simulink model "final_simulation"  (R2023b)
settings: Solver=VariableStepAuto  StartTime=0.0  StopTime=300  RelTol=1e-3
values from neighbouring files (symbols this model uses):
  omega = v/R    [parameters.m]
  R = R1(3)    [parameters.m]
libraries: slpidlib x3
settings Model: Creator=swara  LastModifiedBy=muthu

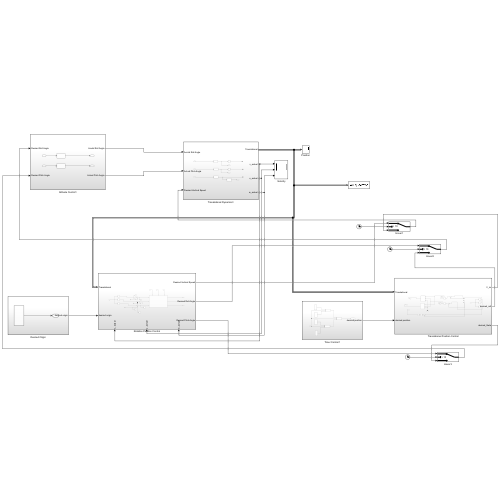
[thumbnail: Simulink's stored preview of the top-level diagram]
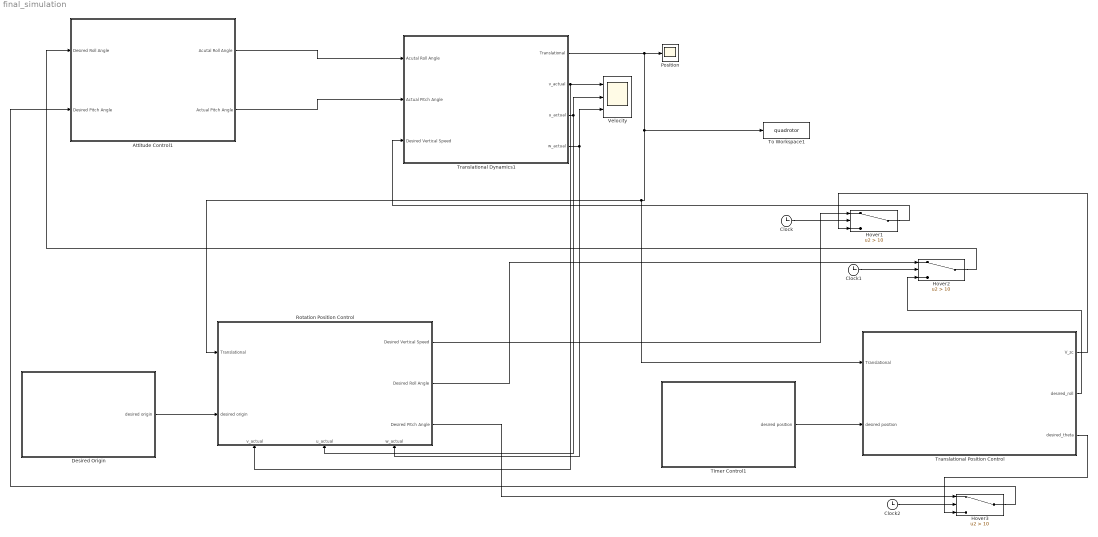
== system final_simulation ==
  Attitude Control1 : Subsystem
  Clock : Clock
  Clock1 : Clock
  Clock2 : Clock
  Desired Origin : Subsystem
  Hover1 : Switch  Criteria=u2 > Threshold  Threshold=10  SaturateOnIntegerOverflow=off  InputSameDT=off
  Hover2 : Switch  Criteria=u2 > Threshold  Threshold=10  SaturateOnIntegerOverflow=off  InputSameDT=off
  Hover3 : Switch  Criteria=u2 > Threshold  Threshold=10  SaturateOnIntegerOverflow=off  InputSameDT=off
  Position : Scope
  Rotation Position Control : Subsystem
      settings: PortSchema="{\"entries\":[{\"content\":{\"sides\":[{\"content\":{\"connectorIds\":[\"In1\",\"In2\"]},\"type\":\"ConnectorPlacement.EquallySpacedRectSide\",\"uuid\":\"b1b3e56e-3c02-4468-8ff7-9257e5b5e807\"},{\"content\":{\"connectorIds\":[\"Out1\",\"Out2\",\"Out3\"],\"side\":\"RIGHT\"},\"type\":\"ConnectorPlacement.EquallySpacedRectSide\",\"uuid\":\"224505eb-429b-4f4e-9eff-5e9145824b2b\"},{\"content\":{\"side\":\"TOP\"},\"type\":\"ConnectorPlacement.EquallySpacedRectSide\",\"uuid\":\"ae18805e-693a-4e7d-a4f9-b6e57170d54a\"},{\"content\":{\"connectorIds\":[\"In3\",\"In4\",\"In5\"],\"side\":\"BOTTOM\"},\"type\":\"ConnectorPlacement.EquallySpacedRectSide\",\"uuid\":\"834ddea8-6bbf-46e8-a21e-4332498dde7e\"}]},\"type\":\"ConnectorPlacement.EquallySpacedConnector\",\"uuid\":\"d1940db1-47fe-4a33-8f26-436ca695897e\"}],\"packageUris\":[\"http://schema.mathworks.com/mf0/Connector/R2020b\"],\"version\":\"1.0\"}"
  Timer Control1 : Subsystem
  To Workspace1 : ToWorkspace  VariableName=quadrotor  SampleTime=-1
  Translational Dynamics1 : Subsystem
  Translational Position Control : Subsystem
  Velocity : Scope  NumInputPorts=3
  wires:
  Attitude Control1/2(Actual Pitch Angle) -> Translational Dynamics1/2(Actual Pitch Angle)
  Translational Dynamics1/2(v_actual) -> Rotation Position Control/3(v_actual), Velocity/1
  Translational Dynamics1/3(u_actual) -> Rotation Position Control/4(u_actual), Velocity/2
  Translational Dynamics1/4(w_actual) -> Rotation Position Control/5(w_actual), Velocity/3
  Translational Dynamics1/1(Translational) -> Position/1, To Workspace1/1, Translational Position Control/1(Translational), Rotation Position Control/1(Translational)
  Attitude Control1/1(Acutal Roll Angle) -> Translational Dynamics1/1(Acutal Roll Angle)
  Desired Origin/1(desired origin) -> Rotation Position Control/2(desired origin)
  Translational Position Control/1(V_zc) -> Hover1/3
  Rotation Position Control/1(Desired Vertical Speed) -> Hover1/1
  Clock/1 -> Hover1/2
  Translational Position Control/2(desired_roll) -> Hover2/3
  Hover2/1 -> Attitude Control1/1(Desired Roll Angle)
  Rotation Position Control/2(Desired Roll Angle) -> Hover2/1
  Clock1/1 -> Hover2/2
  Translational Position Control/3(desired_theta) -> Hover3/3
  Rotation Position Control/3(Desired Pitch Angle) -> Hover3/1
  Clock2/1 -> Hover3/2
  Hover3/1 -> Attitude Control1/2(Desired Pitch Angle)
  Hover1/1 -> Translational Dynamics1/3(Desired Vertical Speed)
  Timer Control1/1(desired position) -> Translational Position Control/2(desired position)

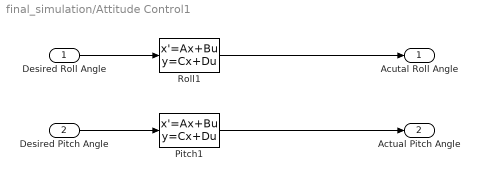
== system final_simulation/Attitude Control1 ==
  Desired Roll Angle : Inport
  Desired Pitch Angle : Inport  Port=2
  Pitch1 : StateSpace  A=[-3.9784 -2.9796; 4 0]  B=[2;0]  C=[1.2569 0.6083]  D=[0]  InitialCondition=0
  Roll1 : StateSpace  A=[-4.2683 -3.1716; 4 0]  B=[2;0]  C=[0.7417 0.4405]  D=[0]  InitialCondition=0
  Acutal Roll Angle : Outport
  Actual Pitch Angle : Outport  Port=2
  wires:
  Pitch1/1 -> Actual Pitch Angle/1
  Desired Pitch Angle/1 -> Pitch1/1
  Roll1/1 -> Acutal Roll Angle/1
  Desired Roll Angle/1 -> Roll1/1

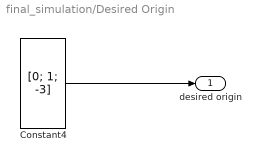
== system final_simulation/Desired Origin ==
  Constant4 : Constant  Value=[0; 1; -3]  VectorParams1D=off
  desired origin : Outport
  wires:
  Constant4/1 -> desired origin/1

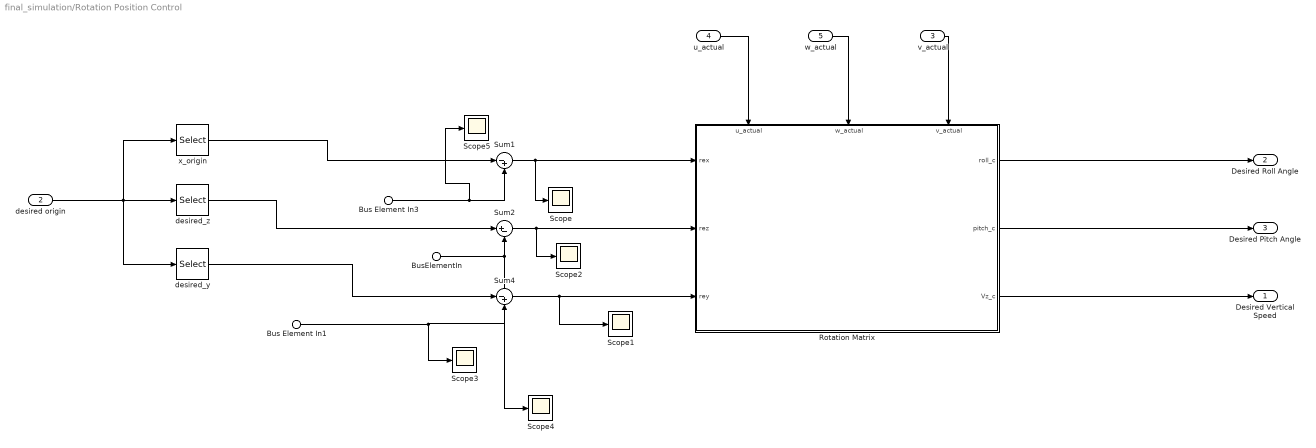
== system final_simulation/Rotation Position Control ==
  Bus Element In3 : Inport  PortName=Translational  Element=x_actual
  Bus Element In1 : Inport  PortName=Translational  Element=y_actual
  BusElementIn : Inport  PortName=Translational  Element=z_actual
  desired origin : Inport  Port=2
  v_actual : Inport  Port=3
  u_actual : Inport  Port=4
  w_actual : Inport  Port=5
  Rotation Matrix : Subsystem
      settings: PortSchema="{\"entries\":[{\"content\":{\"sides\":[{\"content\":{\"connectorIds\":[\"In1\",\"In2\",\"In3\"]},\"type\":\"ConnectorPlacement.EquallySpacedRectSide\",\"uuid\":\"851a648d-3d1b-4670-bb4b-4c1955b2d06c\"},{\"content\":{\"connectorIds\":[\"Out1\",\"Out2\",\"Out3\"],\"side\":\"RIGHT\"},\"type\":\"ConnectorPlacement.EquallySpacedRectSide\",\"uuid\":\"65ea146c-4b0b-429e-8e5f-57ab875054bb\"},{\"content\":{\"connectorIds\":[\"In4\",\"In5\",\"In6\"],\"side\":\"TOP\"},\"type\":\"ConnectorPlacement.EquallySpacedRectSide\",\"uuid\":\"0e78a648-e7f5-443e-b826-3dd94fb81bb4\"}]},\"type\":\"ConnectorPlacement.EquallySpacedConnector\",\"uuid\":\"33f91bbb-2c3f-4173-9364-ab3cef05faeb\"}],\"packageUris\":[\"http://schema.mathworks.com/mf0/Connector/R2020b\"],\"version\":\"1.0\"}"
  Scope{,1..5} (6 alike) : Scope
  Sum1 : Sum  Inputs=|-+
  Sum2 : Sum  Inputs=|+-
  Sum4 : Sum  Inputs=|-+
  desired_y : Selector  InputPortWidth=3  IndexOptions=Index vector (dialog)  Indices=[2]  OutputSizes=1
  desired_z : Selector  InputPortWidth=3  IndexOptions=Index vector (dialog)  Indices=[3]  OutputSizes=1
  x_origin : Selector  InputPortWidth=3  IndexOptions=Index vector (dialog)  Indices=[1]  OutputSizes=1
  Desired Vertical Speed : Outport
  Desired Roll Angle : Outport  Port=2
  Desired Pitch Angle : Outport  Port=3
  wires:
  Sum4/1 -> Scope1/1, Rotation Matrix/3(rey)
  x_origin/1 -> Sum1/1
  desired_y/1 -> Sum4/1
  desired_z/1 -> Sum2/1
  Sum2/1 -> Scope2/1, Rotation Matrix/2(rez)
  Rotation Matrix/1(roll_c) -> Desired Roll Angle/1
  Rotation Matrix/2(pitch_c) -> Desired Pitch Angle/1
  Rotation Matrix/3(Vz_c) -> Desired Vertical Speed/1
  BusElementIn/1 -> Scope4/1, Sum2/2
  v_actual/1 -> Rotation Matrix/6(v_actual)
  u_actual/1 -> Rotation Matrix/4(u_actual)
  w_actual/1 -> Rotation Matrix/5(w_actual)
  Sum1/1 -> Scope/1, Rotation Matrix/1(rex)
  Bus Element In3/1 -> Scope5/1, Sum1/2
  Bus Element In1/1 -> Scope3/1, Sum4/2
  desired origin/1 -> x_origin/1, desired_z/1, desired_y/1

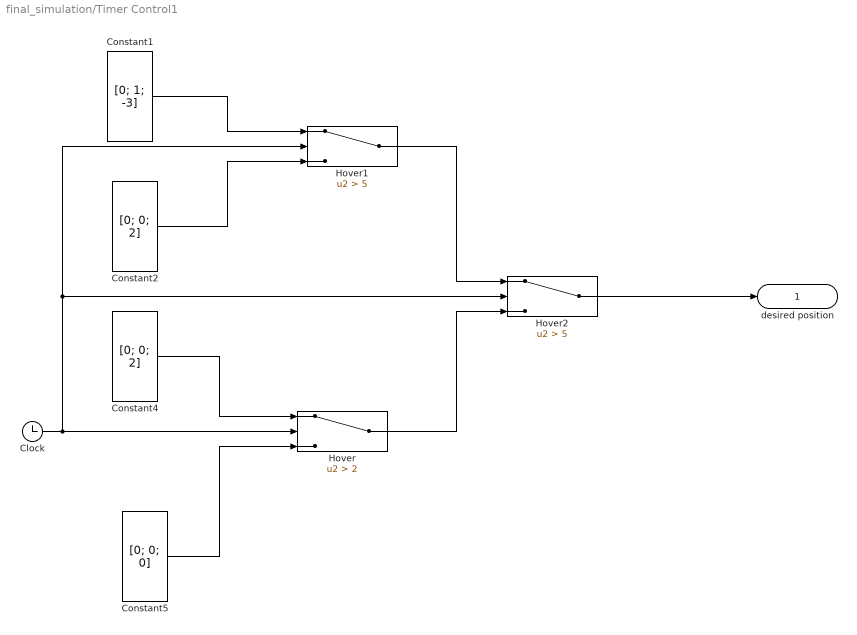
== system final_simulation/Timer Control1 ==
  Clock : Clock
  Constant1 : Constant  Value=[0; 1; -3]  VectorParams1D=off
  Constant2 : Constant  Value=[0; 0; 2]  VectorParams1D=off
  Constant4 : Constant  Value=[0; 0; 2]  VectorParams1D=off
  Constant5 : Constant  Value=[0; 0; 0]  VectorParams1D=off
  Hover : Switch  Criteria=u2 > Threshold  Threshold=2  SaturateOnIntegerOverflow=off  InputSameDT=off
  Hover1 : Switch  Criteria=u2 > Threshold  Threshold=5  SaturateOnIntegerOverflow=off  InputSameDT=off
  Hover2 : Switch  Criteria=u2 > Threshold  Threshold=5  SaturateOnIntegerOverflow=off  InputSameDT=off
  desired position : Outport
  wires:
  Hover1/1 -> Hover2/1
  Hover2/1 -> desired position/1
  Hover/1 -> Hover2/3
  Constant1/1 -> Hover1/1
  Constant2/1 -> Hover1/3
  Clock/1 -> Hover1/2, Hover2/2, Hover/2
  Constant5/1 -> Hover/3
  Constant4/1 -> Hover/1

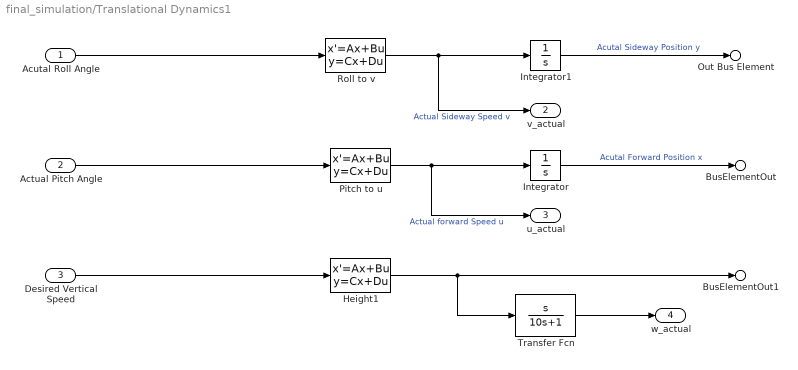
== system final_simulation/Translational Dynamics1 ==
  Acutal Roll Angle : Inport
  Actual Pitch Angle : Inport  Port=2
  Desired Vertical Speed : Inport  Port=3
  Height1 : StateSpace  A=[-5.82 -0.0000036046; 0.0000038147 0]  B=[1024;0]  C=[0.000014907 1319.1]  D=0  InitialCondition=0
  Integrator : Integrator
  Integrator1 : Integrator
  Pitch to u : StateSpace  A=[-0.665]  B=[2]  C=[-3.0772]  D=[0]  InitialCondition=0
  Roll to v : StateSpace  A=[-0.4596]  B=[2]  C=[2.3868]  D=[0]  InitialCondition=0
  Transfer Fcn : TransferFcn  Numerator=[1 0]  Denominator=[10 1]
  Out Bus Element : Outport  PortName=Translational  Element=y_actual
  BusElementOut : Outport  PortName=Translational  Element=x_actual
  BusElementOut1 : Outport  PortName=Translational  Element=z_actual
  v_actual : Outport  Port=2
  u_actual : Outport  Port=3
  w_actual : Outport  Port=4
  wires:
  Height1/1 -> Transfer Fcn/1, BusElementOut1/1
  Desired Vertical Speed/1 -> Height1/1
  Acutal Roll Angle/1 -> Roll to v/1
  Actual Pitch Angle/1 -> Pitch to u/1
  Integrator1/1 -> Out Bus Element/1  "Acutal Sideway Position y"
  Roll to v/1 -> v_actual/1, Integrator1/1  "Actual Sideway Speed v"
  Pitch to u/1 -> u_actual/1, Integrator/1  "Actual forward Speed u"
  Integrator/1 -> BusElementOut/1  "Acutal Forward Position x"
  Transfer Fcn/1 -> w_actual/1

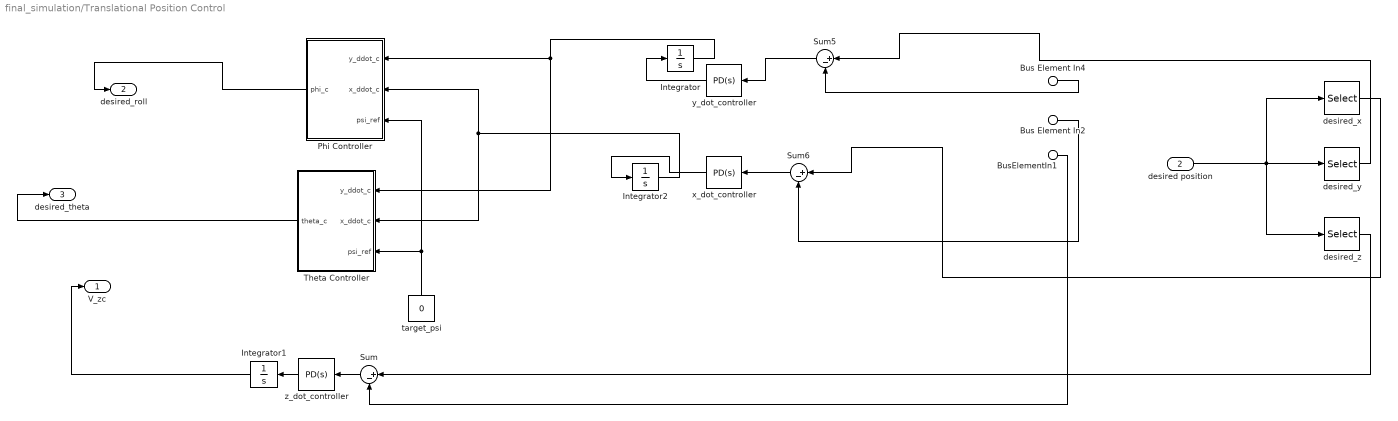
== system final_simulation/Translational Position Control ==
  Bus Element In2 : Inport  PortName=Translational  Element=x_actual
  Bus Element In4 : Inport  PortName=Translational  Element=y_actual
  BusElementIn1 : Inport  PortName=Translational  Element=z_actual
  desired position : Inport  Port=2
  Integrator : Integrator
  Integrator1 : Integrator
  Integrator2 : Integrator
  Phi Controller : Subsystem
  Sum : Sum  Inputs=|+-
  Sum5 : Sum  Inputs=|+-
  Sum6 : Sum  Inputs=|+-
  Theta Controller : Subsystem
  desired_x : Selector  InputPortWidth=3  IndexOptions=Index vector (dialog)  Indices=[1]  OutputSizes=1
  desired_y : Selector  InputPortWidth=3  IndexOptions=Index vector (dialog)  Indices=[2]  OutputSizes=1
  desired_z : Selector  InputPortWidth=3  IndexOptions=Index vector (dialog)  Indices=[3]  OutputSizes=1
  target_psi : Constant  Value=0
  x_dot_controller : slpidlib/PID Controller  Controller=PD  Form=Parallel  TimeDomain=Continuous-time  UseExternalTs=off  SampleTime=-1  IntegratorMethod=Forward Euler  FilterMethod=Forward Euler  ControllerParametersSource=internal  P=0.000973164818719708  I=10  UseKiTs=off  D=0.547582496129018  N=23.2094749491002  UseFilter=on  TunerSelectOption=Transfer Function Based (PID Tuner App)  InitialConditionSource=internal  InitialConditionForIntegrator=0  InitialConditionForFilter=0  DifferentiatorICPrevScaledInput=0  ExternalReset=none  TrackingMode=off  Kt=1  LimitOutput=off  SatLimitsSource=internal  UpperSaturationLimit=inf  LowerSaturationLimit=-inf  LinearizeAsGain=on  AntiWindupMode=none  Kb=1  LimitIntegrator=off  UpperIntegratorSaturationLimit=inf  LowerIntegratorSaturationLimit=-inf  POutMin=[]  POutMax=[]  IOutMin=[]  IOutMax=[]  DOutMin=[]  DOutMax=[]  NOutMin=[]  NOutMax=[]  SumOutMin=[]  SumOutMax=[]  SaturationOutMin=[]  SaturationOutMax=[]  PParamMin=[]  PParamMax=[]  IParamMin=[]  IParamMax=[]  DParamMin=[]  DParamMax=[]  NParamMin=[]  NParamMax=[]  KbParamMin=[]  KbParamMax=[]  KtParamMin=[]  KtParamMax=[]  KbOutMin=[]  KbOutMax=[]  KtOutMin=[]  KtOutMax=[]  IntegratorOutMin=[]  IntegratorOutMax=[]  FilterOutMin=[]  FilterOutMax=[]  SumI1OutMin=[]  SumI1OutMax=[]  SumI2OutMin=[]  SumI2OutMax=[]  SumI3OutMin=[]  SumI3OutMax=[]  SumI4OutMin=[]  SumI4OutMax=[]  SumDOutMin=[]  SumDOutMax=[]  DifferentiatorOutMin=[]  DifferentiatorOutMax=[]  FilterDiffOutCoefMin=[]  FilterDiffOutCoefMax=[]  ReciprocalOutMin=[]  ReciprocalOutMax=[]  SumDenOutMin=[]  SumDenOutMax=[]  SumNumOutMin=[]  SumNumOutMax=[]  DivideOutMin=[]  DivideOutMax=[]  UdiffTsProdOutMin=[]  UdiffTsProdOutMax=[]  NTsProdOutMin=[]  NTsProdOutMax=[]  UintegralTsProdOutMin=[]  UintegralTsProdOutMax=[]  UngainTsProdOutMin=[]  UngainTsProdOutMax=[]  ClampingZeroOutDataTypeStr=Inherit: Inherit via back propagation  ClampingZeroOutMin=[]  ClampingZeroOutMax=[]  FilterDenConstantOutDataTypeStr=Inherit: Inherit via back propagation  FilterDenConstantOutMin=[]  FilterDenConstantOutMax=[]  PCopyOutDataTypeStr=Inherit: Inherit via back propagation  PCopyOutMin=[]  PCopyOutMax=[]  NCopyOutDataTypeStr=Inherit: Inherit via back propagation  NCopyOutMin=[]  NCopyOutMax=[]  IntegratorContinuousStateAttributes=''  IntegratorStateMustResolveToSignalObject=off  IntegratorRTWStateStorageClass=Auto  FilterContinuousStateAttributes=''  FilterStateMustResolveToSignalObject=off  FilterRTWStateStorageClass=Auto  ParallelPVariant=InternalParameters  IdealPVariant=Disabled  IVariant=Disabled  DVariant=InternalParameters  IntegratorVariant=Disabled  SatVariant=Disabled  AWVariant=Disabled  PCopyVariant=Disabled  TRVariant=Disabled  FdbkBlocksVariant=Forward  IdealPFdbkVariant=Disabled  SatFdbkVariant=Disabled  DerivativeFilterVariant=ContFilter  NVariant=InternalParameters  NCopyVariant=Disabled  FilterICVariant=InternalICsFilter  IntegratorICVariant=Disabled  ExternalResetVariant=Disabled  TRSumVariant=Passthrough  SumFdbkVariant=Disabled  SumVariant=Sum_PD  TsampFilterVariant=InternalTs  TsampNgainVariant=Passthrough  TsampIntegralVariant=Disabled_SignalSpec  ExternalSaturationOutDataTypeStr=Inherit: Same as second input
  y_dot_controller : slpidlib/PID Controller  Controller=PD  Form=Parallel  TimeDomain=Continuous-time  UseExternalTs=off  SampleTime=-1  IntegratorMethod=Forward Euler  FilterMethod=Forward Euler  ControllerParametersSource=internal  P=0.390400736412338878  I=10  UseKiTs=off  D=0.400269327887123  N=13.0747973581782  UseFilter=on  TunerSelectOption=Transfer Function Based (PID Tuner App)  InitialConditionSource=internal  InitialConditionForIntegrator=0  InitialConditionForFilter=0  DifferentiatorICPrevScaledInput=0  ExternalReset=none  TrackingMode=off  Kt=1  LimitOutput=off  SatLimitsSource=internal  UpperSaturationLimit=inf  LowerSaturationLimit=-inf  LinearizeAsGain=on  AntiWindupMode=none  Kb=1  LimitIntegrator=off  UpperIntegratorSaturationLimit=inf  LowerIntegratorSaturationLimit=-inf  POutMin=[]  POutMax=[]  IOutMin=[]  IOutMax=[]  DOutMin=[]  DOutMax=[]  NOutMin=[]  NOutMax=[]  SumOutMin=[]  SumOutMax=[]  SaturationOutMin=[]  SaturationOutMax=[]  PParamMin=[]  PParamMax=[]  IParamMin=[]  IParamMax=[]  DParamMin=[]  DParamMax=[]  NParamMin=[]  NParamMax=[]  KbParamMin=[]  KbParamMax=[]  KtParamMin=[]  KtParamMax=[]  KbOutMin=[]  KbOutMax=[]  KtOutMin=[]  KtOutMax=[]  IntegratorOutMin=[]  IntegratorOutMax=[]  FilterOutMin=[]  FilterOutMax=[]  SumI1OutMin=[]  SumI1OutMax=[]  SumI2OutMin=[]  SumI2OutMax=[]  SumI3OutMin=[]  SumI3OutMax=[]  SumI4OutMin=[]  SumI4OutMax=[]  SumDOutMin=[]  SumDOutMax=[]  DifferentiatorOutMin=[]  DifferentiatorOutMax=[]  FilterDiffOutCoefMin=[]  FilterDiffOutCoefMax=[]  ReciprocalOutMin=[]  ReciprocalOutMax=[]  SumDenOutMin=[]  SumDenOutMax=[]  SumNumOutMin=[]  SumNumOutMax=[]  DivideOutMin=[]  DivideOutMax=[]  UdiffTsProdOutMin=[]  UdiffTsProdOutMax=[]  NTsProdOutMin=[]  NTsProdOutMax=[]  UintegralTsProdOutMin=[]  UintegralTsProdOutMax=[]  UngainTsProdOutMin=[]  UngainTsProdOutMax=[]  ClampingZeroOutDataTypeStr=Inherit: Inherit via back propagation  ClampingZeroOutMin=[]  ClampingZeroOutMax=[]  FilterDenConstantOutDataTypeStr=Inherit: Inherit via back propagation  FilterDenConstantOutMin=[]  FilterDenConstantOutMax=[]  PCopyOutDataTypeStr=Inherit: Inherit via back propagation  PCopyOutMin=[]  PCopyOutMax=[]  NCopyOutDataTypeStr=Inherit: Inherit via back propagation  NCopyOutMin=[]  NCopyOutMax=[]  IntegratorContinuousStateAttributes=''  IntegratorStateMustResolveToSignalObject=off  IntegratorRTWStateStorageClass=Auto  FilterContinuousStateAttributes=''  FilterStateMustResolveToSignalObject=off  FilterRTWStateStorageClass=Auto  ParallelPVariant=InternalParameters  IdealPVariant=Disabled  IVariant=Disabled  DVariant=InternalParameters  IntegratorVariant=Disabled  SatVariant=Disabled  AWVariant=Disabled  PCopyVariant=Disabled  TRVariant=Disabled  FdbkBlocksVariant=Forward  IdealPFdbkVariant=Disabled  SatFdbkVariant=Disabled  DerivativeFilterVariant=ContFilter  NVariant=InternalParameters  NCopyVariant=Disabled  FilterICVariant=InternalICsFilter  IntegratorICVariant=Disabled  ExternalResetVariant=Disabled  TRSumVariant=Passthrough  SumFdbkVariant=Disabled  SumVariant=Sum_PD  TsampFilterVariant=InternalTs  TsampNgainVariant=Passthrough  TsampIntegralVariant=Disabled_SignalSpec  ExternalSaturationOutDataTypeStr=Inherit: Same as second input
  z_dot_controller : slpidlib/PID Controller  Controller=PD  Form=Parallel  TimeDomain=Continuous-time  UseExternalTs=off  SampleTime=-1  IntegratorMethod=Forward Euler  FilterMethod=Forward Euler  ControllerParametersSource=internal  P=0.3  I=1  UseKiTs=off  D=3  N=100  UseFilter=on  TunerSelectOption=Transfer Function Based (PID Tuner App)  InitialConditionSource=internal  InitialConditionForIntegrator=0  InitialConditionForFilter=0  DifferentiatorICPrevScaledInput=0  ExternalReset=none  TrackingMode=off  Kt=1  LimitOutput=off  SatLimitsSource=internal  UpperSaturationLimit=inf  LowerSaturationLimit=-inf  LinearizeAsGain=on  AntiWindupMode=none  Kb=1  LimitIntegrator=off  UpperIntegratorSaturationLimit=inf  LowerIntegratorSaturationLimit=-inf  POutMin=[]  POutMax=[]  IOutMin=[]  IOutMax=[]  DOutMin=[]  DOutMax=[]  NOutMin=[]  NOutMax=[]  SumOutMin=[]  SumOutMax=[]  SaturationOutMin=[]  SaturationOutMax=[]  PParamMin=[]  PParamMax=[]  IParamMin=[]  IParamMax=[]  DParamMin=[]  DParamMax=[]  NParamMin=[]  NParamMax=[]  KbParamMin=[]  KbParamMax=[]  KtParamMin=[]  KtParamMax=[]  KbOutMin=[]  KbOutMax=[]  KtOutMin=[]  KtOutMax=[]  IntegratorOutMin=[]  IntegratorOutMax=[]  FilterOutMin=[]  FilterOutMax=[]  SumI1OutMin=[]  SumI1OutMax=[]  SumI2OutMin=[]  SumI2OutMax=[]  SumI3OutMin=[]  SumI3OutMax=[]  SumI4OutMin=[]  SumI4OutMax=[]  SumDOutMin=[]  SumDOutMax=[]  DifferentiatorOutMin=[]  DifferentiatorOutMax=[]  FilterDiffOutCoefMin=[]  FilterDiffOutCoefMax=[]  ReciprocalOutMin=[]  ReciprocalOutMax=[]  SumDenOutMin=[]  SumDenOutMax=[]  SumNumOutMin=[]  SumNumOutMax=[]  DivideOutMin=[]  DivideOutMax=[]  UdiffTsProdOutMin=[]  UdiffTsProdOutMax=[]  NTsProdOutMin=[]  NTsProdOutMax=[]  UintegralTsProdOutMin=[]  UintegralTsProdOutMax=[]  UngainTsProdOutMin=[]  UngainTsProdOutMax=[]  ClampingZeroOutDataTypeStr=Inherit: Inherit via back propagation  ClampingZeroOutMin=[]  ClampingZeroOutMax=[]  FilterDenConstantOutDataTypeStr=Inherit: Inherit via back propagation  FilterDenConstantOutMin=[]  FilterDenConstantOutMax=[]  PCopyOutDataTypeStr=Inherit: Inherit via back propagation  PCopyOutMin=[]  PCopyOutMax=[]  NCopyOutDataTypeStr=Inherit: Inherit via back propagation  NCopyOutMin=[]  NCopyOutMax=[]  IntegratorContinuousStateAttributes=''  IntegratorStateMustResolveToSignalObject=off  IntegratorRTWStateStorageClass=Auto  FilterContinuousStateAttributes=''  FilterStateMustResolveToSignalObject=off  FilterRTWStateStorageClass=Auto  ParallelPVariant=InternalParameters  IdealPVariant=Disabled  IVariant=Disabled  DVariant=InternalParameters  IntegratorVariant=Disabled  SatVariant=Disabled  AWVariant=Disabled  PCopyVariant=Disabled  TRVariant=Disabled  FdbkBlocksVariant=Forward  IdealPFdbkVariant=Disabled  SatFdbkVariant=Disabled  DerivativeFilterVariant=ContFilter  NVariant=InternalParameters  NCopyVariant=Disabled  FilterICVariant=InternalICsFilter  IntegratorICVariant=Disabled  ExternalResetVariant=Disabled  TRSumVariant=Passthrough  SumFdbkVariant=Disabled  SumVariant=Sum_PD  TsampFilterVariant=InternalTs  TsampNgainVariant=Passthrough  TsampIntegralVariant=Disabled_SignalSpec  ExternalSaturationOutDataTypeStr=Inherit: Same as second input
  V_zc : Outport
  desired_roll : Outport  Port=2
  desired_theta : Outport  Port=3
  wires:
  y_dot_controller/1 -> Integrator/1
  desired position/1 -> desired_z/1, desired_x/1, desired_y/1
  target_psi/1 -> Phi Controller/3(psi_ref), Theta Controller/3(psi_ref)
  z_dot_controller/1 -> Integrator1/1
  Sum5/1 -> y_dot_controller/1
  x_dot_controller/1 -> Integrator2/1
  Sum6/1 -> x_dot_controller/1
  Sum/1 -> z_dot_controller/1
  Bus Element In2/1 -> Sum6/2
  Integrator2/1 -> Theta Controller/2(x_ddot_c), Phi Controller/2(x_ddot_c)
  desired_y/1 -> Sum5/1
  Integrator/1 -> Theta Controller/1(y_ddot_c), Phi Controller/1(y_ddot_c)
  Bus Element In4/1 -> Sum5/2
  desired_x/1 -> Sum6/1
  desired_z/1 -> Sum/1
  BusElementIn1/1 -> Sum/2
  Phi Controller/1(phi_c) -> desired_roll/1
  Theta Controller/1(theta_c) -> desired_theta/1
  Integrator1/1 -> V_zc/1

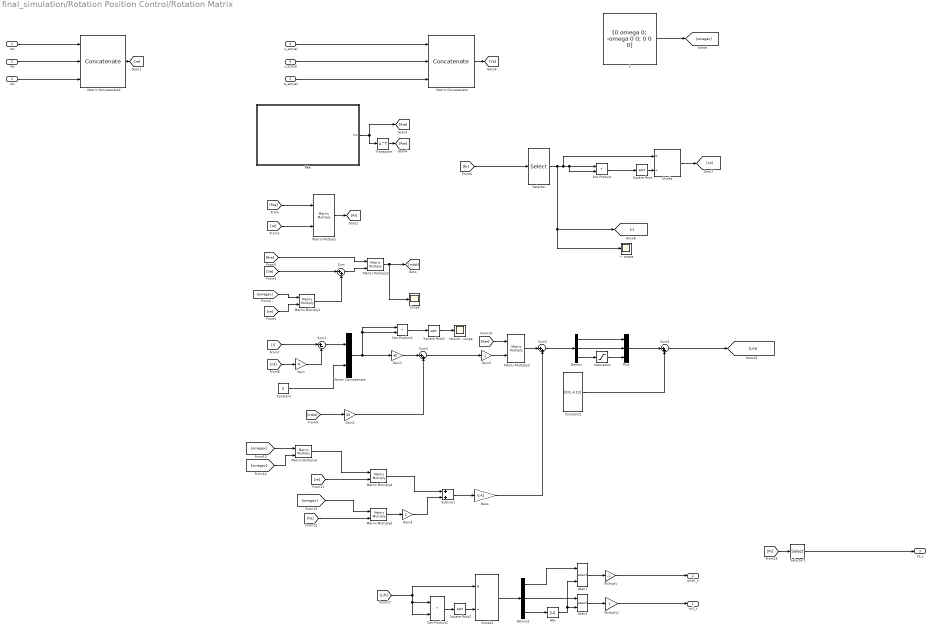
== system final_simulation/Rotation Position Control/Rotation Matrix ==
  rex : Inport
  rez : Inport  Port=2
  rey : Inport  Port=3
  u_actual : Inport  Port=4
  w_actual : Inport  Port=5
  v_actual : Inport  Port=6
  1 : Constant  Value=[0 omega 0; -omega 0 0; 0 0 0]  VectorParams1D=off
  Abs : Abs  SaturateOnIntegerOverflow=off
  Atan1 : Trigonometry  Operator=atan2
  Atan2 : Trigonometry  Operator=atan2
  Constant : Constant  Value=0
  Constant2 : Constant  Value=[0;0;-4.12]  VectorParams1D=off
  Demux : Demux  Outputs=3
  Demux1 : Demux  Outputs=3
  Divide : Product  Inputs=*/
  Divide1 : Product  Inputs=*/
  Dot Product : DotProduct  OutDataTypeStr=Inherit: Inherit via internal rule
  Dot Product1 : DotProduct  OutDataTypeStr=Inherit: Inherit via internal rule
  Dot Product2 : DotProduct  OutDataTypeStr=Inherit: Inherit via internal rule
  Gain : Gain  Gain=R
  Gain1 : Gain  Gain=40
  Gain2 : Gain  Gain=30
  Gain3 : Gain  Gain=-1
  Gain4 : Gain  Gain=2
  Mass : Gain  Gain=0.42
  Matrix Concatenate : Concatenate  NumInputs=3  Mode=Multidimensional array
  Matrix Concatenate2 : Concatenate  NumInputs=3  Mode=Multidimensional array
  Matrix Multiply{,1..6} (7 alike) : Product  Multiplication=Matrix(*)
  Multiply : Gain  Gain=-1
  Multiply1 : Gain
  Mux : Mux  Inputs=3
  RRe : Subsystem
  Saturation : Saturate
  Scope : Scope
  Selector : Selector  InputPortWidth=3  IndexOptions=Index vector (dialog)  Indices=[1 2]  OutputSizes=1
  Selector1 : Selector  InputPortWidth=3  IndexOptions=Index vector (dialog)  Indices=[3]  OutputSizes=1
  Square Root : Sqrt
  Square Root1 : Sqrt
  Square Root2 : Sqrt
  Subtract : Sum
  Sum{,2..4} (4 alike) : Sum  Inputs=|++
  Sum1 : Sum  Inputs=|+-
  Transpose : Math  Operator=transpose  SignedPower=on
  Vector Concatenate : Concatenate
  r - scope : Scope
  rdnorm - scope : Scope
  roll_c : Outport
  pitch_c : Outport  Port=2
  Vz_c : Outport  Port=3
  wires:
  rex/1 -> Matrix Concatenate2/1
  RRe/1(RdI) -> Transpose/1, [Rre]
  Transpose/1 -> [Rer]
  [Rre] -> Matrix Multiply/1
  [re] -> Matrix Multiply/2
  Matrix Multiply/1 -> [Rr]
  u_actual/1 -> Matrix Concatenate/1
  v_actual/1 -> Matrix Concatenate/2
  rey/1 -> Matrix Concatenate2/2
  Matrix Concatenate/1 -> [Ve]
  [omegax] -> Matrix Multiply1/1
  [re] -> Matrix Multiply1/2
  Matrix Multiply1/1 -> Sum/2
  [Ve] -> Sum/1
  Sum/1 -> Matrix Multiply2/2
  [Rre] -> Matrix Multiply2/1
  Matrix Multiply2/1 -> Scope/1, [rrdot]
  1/1 -> [omegax]
  Square Root/1 -> Divide/2
  Divide/1 -> [n2]
  [n2] -> Gain/1
  [r] -> Sum1/1
  Gain/1 -> Sum1/2
  Sum1/1 -> Vector Concatenate/1
  Constant/1 -> Vector Concatenate/2
  Vector Concatenate/1 -> Dot Product1/1, Dot Product1/2, Gain1/1
  Dot Product1/1 -> Square Root1/1
  [rrdot] -> Gain2/1
  Gain1/1 -> Sum2/1
  Gain2/1 -> Sum2/2
  Sum2/1 -> Gain3/1
  Gain3/1 -> Matrix Multiply3/2
  [Rer] -> Matrix Multiply3/1
  Matrix Multiply3/1 -> Sum3/1
  [omegax] -> Matrix Multiply5/1
  Gain4/1 -> Subtract/2
  [re] -> Matrix Multiply4/2
  Matrix Multiply5/1 -> Gain4/1
  Matrix Multiply4/1 -> Subtract/1
  Subtract/1 -> Mass/1
  Matrix Multiply6/1 -> Matrix Multiply4/1
  [omegax] -> Matrix Multiply6/1
  [omegax] -> Matrix Multiply6/2
  [Ve] -> Matrix Multiply5/2
  Mass/1 -> Sum3/2
  Sum3/1 -> Demux/1
  Demux/1 -> Mux/1
  Demux/2 -> Mux/2
  Demux/3 -> Saturation/1
  Saturation/1 -> Mux/3
  Mux/1 -> Sum4/1
  Constant2/1 -> Sum4/2
  Sum4/1 -> [Lift]
  Abs/1 -> Atan1/2, Atan2/2
  Dot Product2/1 -> Square Root2/1
  Demux1/1 -> Atan1/1
  Demux1/2 -> Atan2/1
  Square Root2/1 -> Divide1/2
  Atan2/1 -> Multiply1/1
  Demux1/3 -> Abs/1
  [Lift] -> Dot Product2/2, Dot Product2/1, Divide1/1
  Divide1/1 -> Demux1/1
  Atan1/1 -> Multiply/1
  [Rr] -> Selector/1
  rez/1 -> Matrix Concatenate2/3
  w_actual/1 -> Matrix Concatenate/3
  Matrix Concatenate2/1 -> [re]
  Selector/1 -> r - scope/1, [r], Divide/1, Dot Product/2, Dot Product/1
  Dot Product/1 -> Square Root/1
  Multiply/1 -> pitch_c/1
  Multiply1/1 -> roll_c/1
  Selector1/1 -> Vz_c/1
  [Rr] -> Selector1/1
  Square Root1/1 -> rdnorm - scope/1

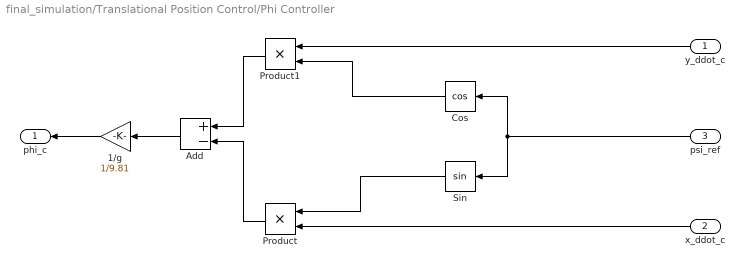
== system final_simulation/Translational Position Control/Phi Controller ==
  y_ddot_c : Inport
  x_ddot_c : Inport  Port=2
  psi_ref : Inport  Port=3
  1/g : Gain  Gain=1/9.81
  Add : Sum  Inputs=+-
  Cos : Trigonometry  Operator=cos
  Product : Product
  Product1 : Product
  Sin : Trigonometry
  phi_c : Outport
  wires:
  Cos/1 -> Product1/2
  Product1/1 -> Add/1
  psi_ref/1 -> Cos/1, Sin/1
  Product/1 -> Add/2
  Add/1 -> 1/g/1
  1/g/1 -> phi_c/1
  Sin/1 -> Product/1
  y_ddot_c/1 -> Product1/1
  x_ddot_c/1 -> Product/2

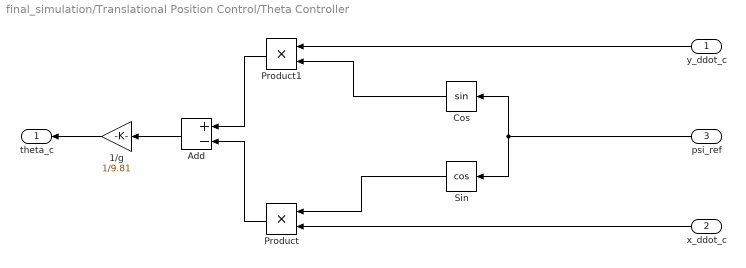
== system final_simulation/Translational Position Control/Theta Controller ==
  y_ddot_c : Inport
  x_ddot_c : Inport  Port=2
  psi_ref : Inport  Port=3
  1/g : Gain  Gain=1/9.81
  Add : Sum  Inputs=+-
  Cos : Trigonometry
  Product : Product
  Product1 : Product
  Sin : Trigonometry  Operator=cos
  theta_c : Outport
  wires:
  Cos/1 -> Product1/2
  Product1/1 -> Add/1
  psi_ref/1 -> Cos/1, Sin/1
  Product/1 -> Add/2
  Add/1 -> 1/g/1
  1/g/1 -> theta_c/1
  Sin/1 -> Product/1
  y_ddot_c/1 -> Product1/1
  x_ddot_c/1 -> Product/2

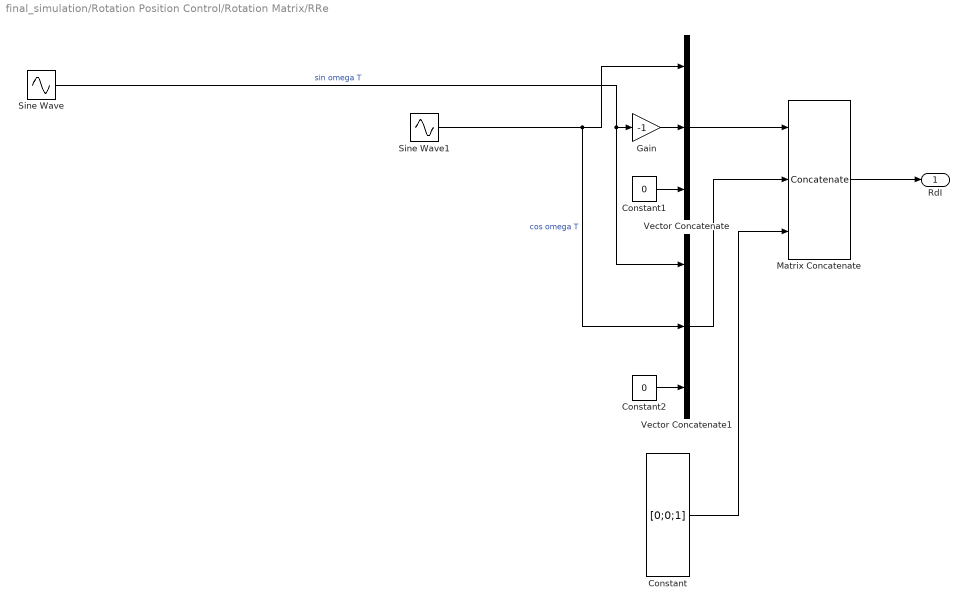
== system final_simulation/Rotation Position Control/Rotation Matrix/RRe ==
  Constant : Constant  Value=[0;0;1]  VectorParams1D=off
  Constant1 : Constant  Value=0  VectorParams1D=off
  Constant2 : Constant  Value=0  VectorParams1D=off
  Gain : Gain  Gain=-1
  Matrix Concatenate : Concatenate  NumInputs=3  Mode=Multidimensional array  ConcatenateDimension=2
  Sine Wave : Sin  Frequency=omega/(2*3.1415)  Phase=-1  SampleTime=0
  Sine Wave1 : Sin  Frequency=omega/(2*pi)  Phase=pi/2 - 1  SampleTime=0
  Vector Concatenate : Concatenate  NumInputs=3
  Vector Concatenate1 : Concatenate  NumInputs=3
  RdI : Outport  VectorParamsAs1DForOutWhenUnconnected=off
  wires:
  Vector Concatenate1/1 -> Matrix Concatenate/2
  Vector Concatenate/1 -> Matrix Concatenate/1
  Constant2/1 -> Vector Concatenate1/3
  Constant1/1 -> Vector Concatenate/3
  Sine Wave/1 -> Vector Concatenate1/1, Gain/1  "sin omega T"
  Constant/1 -> Matrix Concatenate/3
  Sine Wave1/1 -> Vector Concatenate1/2, Vector Concatenate/1  "cos omega T"
  Matrix Concatenate/1 -> RdI/1
  Gain/1 -> Vector Concatenate/2
